simulink model "coverage_model_2019"  (R2019b)
settings: Solver=FixedStepDiscrete  StartTime=0.0  StopTime=50  FixedStep=1  RelTol=1e-3
values from neighbouring files (symbols this model uses):
  Ignition : value not decoded    [ALS_Project_dd.sldd]
  Visual : value not decoded    [ALS_Project_dd.sldd]
undefined symbols (not defined in the file or in its folder): Als_Mode, Corner_Light, sigbuilder_block
libraries: simulink x10
settings Model: NumberOfSteps=2  Creator=hp  LastModifiedBy=hp
settings ConfigComp: CovMetricSettings=dcmwe

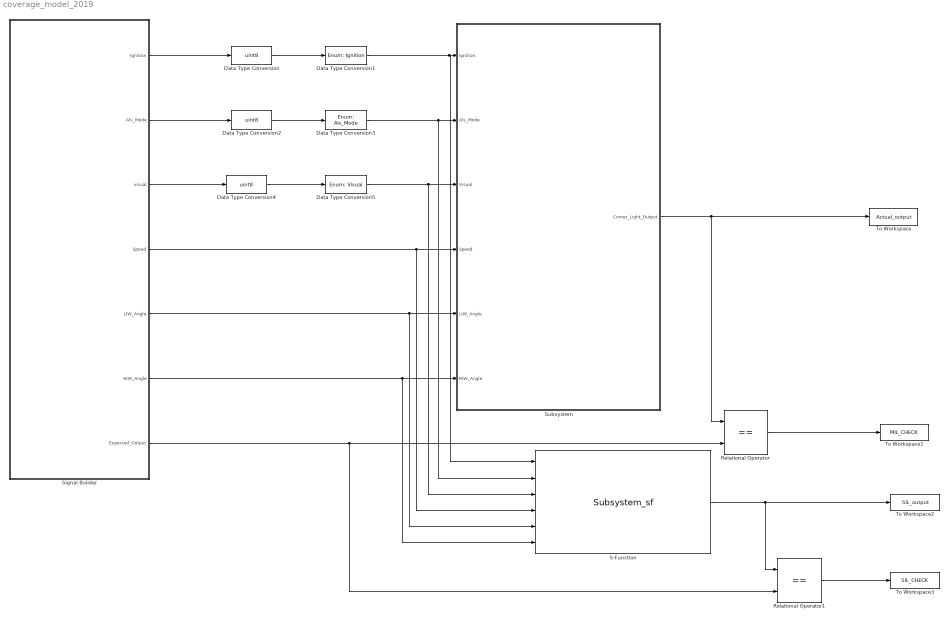
== system coverage_model_2019 ==
  Data Type Conversion : DataTypeConversion  OutDataTypeStr=uint8  SaturateOnIntegerOverflow=on  LockScale=on
  Data Type Conversion1 : DataTypeConversion  OutDataTypeStr=Enum: Ignition  SaturateOnIntegerOverflow=on  LockScale=on
  Data Type Conversion2 : DataTypeConversion  OutDataTypeStr=uint8  SaturateOnIntegerOverflow=on  LockScale=on
  Data Type Conversion3 : DataTypeConversion  OutDataTypeStr=Enum: Als_Mode  SaturateOnIntegerOverflow=on  LockScale=on
  Data Type Conversion4 : DataTypeConversion  OutDataTypeStr=uint8  SaturateOnIntegerOverflow=on  LockScale=on
  Data Type Conversion5 : DataTypeConversion  OutDataTypeStr=Enum: Visual  SaturateOnIntegerOverflow=on  LockScale=on
  Relational Operator : RelationalOperator  Operator===  OutDataTypeStr=boolean  RndMeth=Simplest
  Relational Operator1 : RelationalOperator  Operator===  OutDataTypeStr=boolean  RndMeth=Simplest
  S-Function : S-Function  FunctionName=Subsystem_sf  SFunctionDeploymentMode=off  EnableBusSupport=off
  Signal Builder : Subsystem  Tag=STV Subsys  LoadFcn=sigbuilder_block('load');  StartFcn=sigbuilder_block('start');  StopFcn=sigbuilder_block('stop');  ClipboardFcn=sigbuilder_block('clipboard');  mask(Sigbuilder block){tuvar=[0:10]}
      mask help: Simulink:masks:SigbuilderBlock_MD
      mask init:
      | if ~strcmp(get_param(bdroot(gcbh),'SimulationStatus'),'stopped') tuvar = sigbuilder_block('maskInit'); end
      settings: CopyFcn=sigbuilder_block('copy');  DeleteFcn=sigbuilder_block('delete');  ModelCloseFcn=sigbuilder_block('modelClose');  PreSaveFcn=sigbuilder_block('preSave');  PauseFcn=sigbuilder_block('pause');  ContinueFcn=sigbuilder_block('continue');  NameChangeFcn=sigbuilder_block('namechange');  OpenFcn=sigbuilder_block('open',[437.6 153 550.4 359.25 ]);  CloseFcn=sigbuilder_block('close');
      mask Display: plot(0, 0, 100, 100,[2, 2, 32, 32, 2], [68, 8, 8, 68, 68],[32, 2], [38, 38], [32, 19, 2],[53, 60, 44], [32, 17, 17, 2],[16, 16, 31, 31]);txt = getActiveGroup(gcbh);text(2, 100, txt,'verticalAlignment', 'top');
  Subsystem : Subsystem  TreatAsAtomicUnit=on
  To Workspace : ToWorkspace  VariableName=Actual_output  SaveFormat=Timeseries  SampleTime=-1
  To Workspace1 : ToWorkspace  VariableName=MIL_CHECK  SaveFormat=Timeseries  SampleTime=-1
  To Workspace2 : ToWorkspace  VariableName=SIL_output  SaveFormat=Timeseries  SampleTime=-1
  To Workspace3 : ToWorkspace  VariableName=SIL_CHECK  SaveFormat=Timeseries  SampleTime=-1
  wires:
  Data Type Conversion1/1 -> S-Function/1, Subsystem/1(Ignition)
  Data Type Conversion/1 -> Data Type Conversion1/1
  Data Type Conversion3/1 -> S-Function/2, Subsystem/2(Als_Mode)
  Data Type Conversion2/1 -> Data Type Conversion3/1
  Data Type Conversion4/1 -> Data Type Conversion5/1
  Data Type Conversion5/1 -> S-Function/3, Subsystem/3(Visual)
  Signal Builder/1(Ignition) -> Data Type Conversion/1
  Signal Builder/2(Als_Mode) -> Data Type Conversion2/1
  Signal Builder/3(visual) -> Data Type Conversion4/1
  Signal Builder/4(Speed) -> S-Function/4, Subsystem/4(Speed)
  Signal Builder/5(LIW_Angle) -> S-Function/5, Subsystem/5(LIW_Angle)
  Signal Builder/6(RIW_Angle) -> S-Function/6, Subsystem/6(RIW_Angle)
  Subsystem/1(Corner_Light_Output) -> To Workspace/1, Relational Operator/1
  Signal Builder/7(Expected_Output) -> Relational Operator1/2, Relational Operator/2
  Relational Operator/1 -> To Workspace1/1
  S-Function/1 -> Relational Operator1/1, To Workspace2/1
  Relational Operator1/1 -> To Workspace3/1

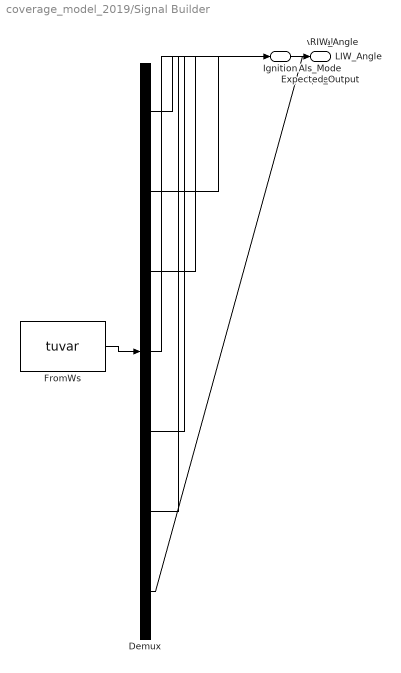
== system coverage_model_2019/Signal Builder ==
  Demux : Demux  Tag=STV Demux  Outputs=7
      settings: DisplayOption=none
  FromWs : FromWorkspace  Tag=STV FromWs  VariableName=tuvar
      SigBuilderData=|
      | common.afterFinalStr = 'Extrapolate'
      | common.sampleTime = 0
      | dataSet.timeRange = [0 47]
      | dataSet.name = 'Sheet1'
      | sbobj.Name = 'Signal Builder'
      | sbobj.Groups.Name = 'Sheet1'
      | sbobj.Groups.Signals(1).Name = 'Ignition'
      | sbobj.Groups.Signals(1).XData = [0 1 2 3 4 5 6 7 8 9 10 11 12 13 14 15 16 17 18 19 20 21 22 23 24 25 26 27 28 29 30 31 32 33 34 35 36 37 38 39 40 41 42 43 44 45 46 47]
      | sbobj.Groups.Signals(1).YData = [0 0 0 0 0 0 0 0 1 1 1 1 1 1 1 1 0 0 0 0 0 0 0 0 1 1 1 1 1 1 1 1 0 0 0 0 0 0 0 0 1 1 1 1 1 1 1 1]
      | sbobj.Groups.Signals(2).Name = 'Als_Mode'
      | sbobj.Groups.Signals(2).XData = [0 1 2 3 4 5 6 7 8 9 10 11 12 13 14 15 16 17 18 19 20 21 22 23 24 25 26 27 28 29 30 31 32 33 34 35 36 37 38 39 40 41 42 43 44 45 46 47]
      | sbobj.Groups.Signals(2).YData = [0 0 0 0 1 1 1 1 0 0 0 0 1 1 1 1 0 0 0 0 1 1 1 1 0 0 0 0 1 1 1 1 0 0 0 0 1 1 1 1 0 0 0 0 1 1 1 1]
      | sbobj.Groups.Signals(3).Name = 'visual'
      | sbobj.Groups.Signals(3).XData = [0 1 2 3 4 5 6 7 8 9 10 11 12 13 14 15 16 17 18 19 20 21 22 23 24 25 26 27 28 29 30 31 32 33 34 35 36 37 38 39 40 41 42 43 44 45 46 47]
      | sbobj.Groups.Signals(3).YData = [0 0 1 1 0 0 1 1 0 0 1 1 0 0 1 1 0 0 1 1 0 0 1 1 0 0 1 1 0 0 1 1 0 0 1 1 0 0 1 1 0 0 1 1 0 0 1 1]
      | sbobj.Groups.Signals(4).Name = 'Speed'
      | sbobj.Groups.Signals(4).XData = [0 1 2 3 4 5 6 7 8 9 10 11 12 13 14 15 16 17 18 19 20 21 22 23 24 25 26 27 28 29 30 31 32 33 34 35 36 37 38 39 40 41 42 43 44 45 46 47]
      | sbobj.Groups.Signals(4).YData = [50 25 50 25 50 25 50 25 50 25 50 25 50 25 50 25 50 50 50 50 50 50 50 50 50 50 50 50 50 50 50 50 50 50 50 50 50 50 50 50 50 50 50 50 50 50 50 50]
      | sbobj.Groups.Signals(5).Name = 'LIW_Angle'
      | sbobj.Groups.Signals(5).XData = [0 1 2 3 4 5 6 7 8 9 10 11 12 13 14 15 16 17 18 19 20 21 22 23 24 25 26 27 28 29 30 31 32 33 34 35 36 37 38 39 40 41 42 43 44 45 46 47]
      | sbobj.Groups.Signals(5).YData = [0 0 0 0 0 0 0 0 0 0 0 0 0 0 0 0 0 7 0 7 0 7 0 7 0 7 0 7 0 7 0 7 0 0 0 0 0 0 0 0 0 0 0 0 0 0 0 0]
      | sbobj.Groups.Signals(6).Name = 'RIW_Angle'
      | sbobj.Groups.Signals(6).XData = [0 1 2 3 4 5 6 7 8 9 10 11 12 13 14 15 16 17 18 19 20 21 22 23 24 25 26 27 28 29 30 31 32 33 34 35 36 37 38 39 40 41 42 43 44 45 46 47]
      | sbobj.Groups.Signals(6).YData = [0 0 0 0 0 0 0 0 0 0 0 0 0 0 0 0 0 0 0 0 0 0 0 0 0 0 0 0 0 0 0 0 0 7 0 7 0 7 0 7 0 7 0 7 0 7 0 7]
      | sbobj.Groups.Signals(7).Name = 'Expected_Output'
      | sbobj.Groups.Signals(7).XData = [0 1 2 3 4 5 6 7 8 9 10 11 12 13 14 15 16 17 18 19 20 21 22 23 24 25 26 27 28 29 30 31 32 33 34 35 36 37 38 39 40 41 42 43 44 45 46 47]
      | sbobj.Groups.Signals(7).YData = [0 0 0 0 0 0 0 0 0 0 0 0 0 0 0 1 0 0 0 0 0 0 0 0 0 0 0 0 0 0 0 2 0 0 0 0 0 0 0 0 0 0 0 0 0 0 0 3]
      | sbobj.Groups.TimeRange = [0 47]
  Ignition : Outport  Tag=STV Outport
  Als_Mode : Outport  Tag=STV Outport  Port=2
  visual : Outport  Tag=STV Outport  Port=3
  Speed : Outport  Tag=STV Outport  Port=4
  LIW_Angle : Outport  Tag=STV Outport  Port=5
  RIW_Angle : Outport  Tag=STV Outport  Port=6
  Expected_Output : Outport  Tag=STV Outport  Port=7
  wires:
  Demux/1 -> Ignition/1
  FromWs/1 -> Demux/1
  Demux/2 -> Als_Mode/1
  Demux/3 -> visual/1
  Demux/4 -> Speed/1
  Demux/5 -> LIW_Angle/1
  Demux/6 -> RIW_Angle/1
  Demux/7 -> Expected_Output/1

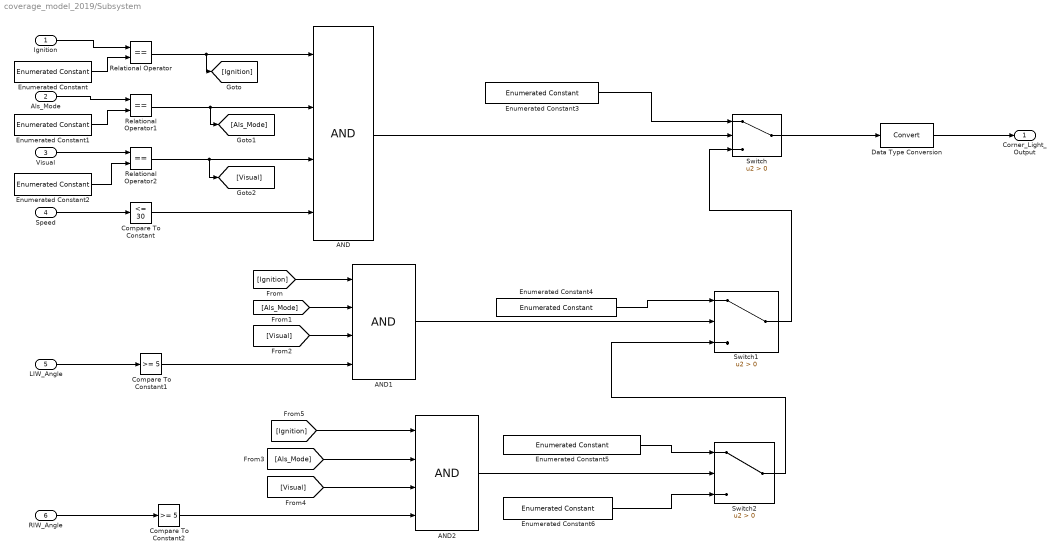
== system coverage_model_2019/Subsystem ==
  Ignition : Inport
  Als_Mode : Inport  Port=2
  Visual : Inport  Port=3
  Speed : Inport  Port=4
  LIW_Angle : Inport  Port=5
  RIW_Angle : Inport  Port=6
  AND : Logic  Inputs=4  AllPortsSameDT=off  OutDataTypeStr=boolean
  AND1 : Logic  Inputs=4  AllPortsSameDT=off  OutDataTypeStr=boolean
  AND2 : Logic  Inputs=4  AllPortsSameDT=off  OutDataTypeStr=boolean
  Compare To Constant : simulink/Logic and Bit Operations/Compare To Constant  relop=<=  const=30  OutDataTypeStr=boolean
  Compare To Constant1 : simulink/Logic and Bit Operations/Compare To Constant  relop=>=  const=5  OutDataTypeStr=boolean
  Compare To Constant2 : simulink/Logic and Bit Operations/Compare To Constant  relop=>=  const=5  OutDataTypeStr=boolean
  Data Type Conversion : DataTypeConversion  SaturateOnIntegerOverflow=on  LockScale=on
  Enumerated Constant : simulink/Sources/Enumerated Constant  OutDataTypeStr=Enum: Ignition  Value=Ignition.Ignition_On  SampleTime=inf
  Enumerated Constant1 : simulink/Sources/Enumerated Constant  OutDataTypeStr=Enum: Als_Mode  Value=Als_Mode.Als__Mode_On  SampleTime=inf
  Enumerated Constant2 : simulink/Sources/Enumerated Constant  OutDataTypeStr=Enum: Visual  Value=Visual.Night_Mode  SampleTime=inf
  Enumerated Constant3 : simulink/Sources/Enumerated Constant  OutDataTypeStr=Enum: Corner_Light  Value=Corner_Light.Corner_Light_On  SampleTime=inf
  Enumerated Constant4 : simulink/Sources/Enumerated Constant  OutDataTypeStr=Enum: Corner_Light  Value=Corner_Light.Left_Corner_Light_On  SampleTime=inf
  Enumerated Constant5 : simulink/Sources/Enumerated Constant  OutDataTypeStr=Enum: Corner_Light  Value=Corner_Light.Right_Corner_Light_On  SampleTime=inf
  Enumerated Constant6 : simulink/Sources/Enumerated Constant  OutDataTypeStr=Enum: Corner_Light  Value=Corner_Light.Corner_Light_Off  SampleTime=inf
  Relational Operator : RelationalOperator  Operator===  OutDataTypeStr=boolean  RndMeth=Simplest
  Relational Operator1 : RelationalOperator  Operator===  OutDataTypeStr=boolean  RndMeth=Simplest
  Relational Operator2 : RelationalOperator  Operator===  OutDataTypeStr=boolean  RndMeth=Simplest
  Switch : Switch  Criteria=u2 > Threshold
  Switch1 : Switch  Criteria=u2 > Threshold
  Switch2 : Switch  Criteria=u2 > Threshold
  Corner_Light_Output : Outport
  wires:
  Switch2/1 -> Switch1/3
  Enumerated Constant1/1 -> Relational Operator1/2
  Compare To Constant1/1 -> AND1/4
  Visual/1 -> Relational Operator2/1
  Compare To Constant2/1 -> AND2/4
  Switch1/1 -> Switch/3
  Relational Operator2/1 -> [Visual], AND/3
  [Ignition] -> AND1/1
  LIW_Angle/1 -> Compare To Constant1/1
  Data Type Conversion/1 -> Corner_Light_Output/1
  AND2/1 -> Switch2/2
  [Visual] -> AND2/3
  Ignition/1 -> Relational Operator/1
  RIW_Angle/1 -> Compare To Constant2/1
  Enumerated Constant3/1 -> Switch/1
  [Visual] -> AND1/3
  AND1/1 -> Switch1/2
  [Als_Mode] -> AND1/2
  AND/1 -> Switch/2
  Enumerated Constant4/1 -> Switch1/1
  Enumerated Constant6/1 -> Switch2/3
  Relational Operator/1 -> [Ignition], AND/1
  Enumerated Constant5/1 -> Switch2/1
  Switch/1 -> Data Type Conversion/1
  Speed/1 -> Compare To Constant/1
  Als_Mode/1 -> Relational Operator1/1
  Relational Operator1/1 -> [Als_Mode], AND/2
  Enumerated Constant/1 -> Relational Operator/2
  [Als_Mode] -> AND2/2
  Enumerated Constant2/1 -> Relational Operator2/2
  Compare To Constant/1 -> AND/4
  [Ignition] -> AND2/1
